simulink model "hcci_eng"  (R2018a)
settings: Solver=VariableStepAuto  StartTime=0.0  StopTime=10.0  RelTol=1e-3
values from neighbouring files (symbols this model uses):
  A01 = ???    [hcci_sim.m]
  A20 = ???    [hcci_sim.m]
  A21 = ???    [hcci_sim.m]
  b1_0 = ???    [load_param.m]
  b2_0 = ???    [load_param.m]
  C_d = ???    [hcci_sim.m]
  dT_er2 = 75    [load_param.m]
  gamma = 1.4    [load_param.m]
  m1_0 = ???    [load_param.m]
  m2_0 = ???    [load_param.m]
  N = 1000    [hcci_sim.m]
  p0 = 1.01    [load_param.m]
  R = 296.25    [load_param.m]
  T1 = 90 + 273.15    (= 363.15)    [load_param.m]
  tau = 120 / N    (= 0.12)    [hcci_sim.m]
  V1 = ???    [load_param.m]
  V2 = ???    [load_param.m]
undefined symbols (not defined in the file or in its folder): p2_0
settings Model: Creator=Lenovo  LastModifiedBy=Lenovo

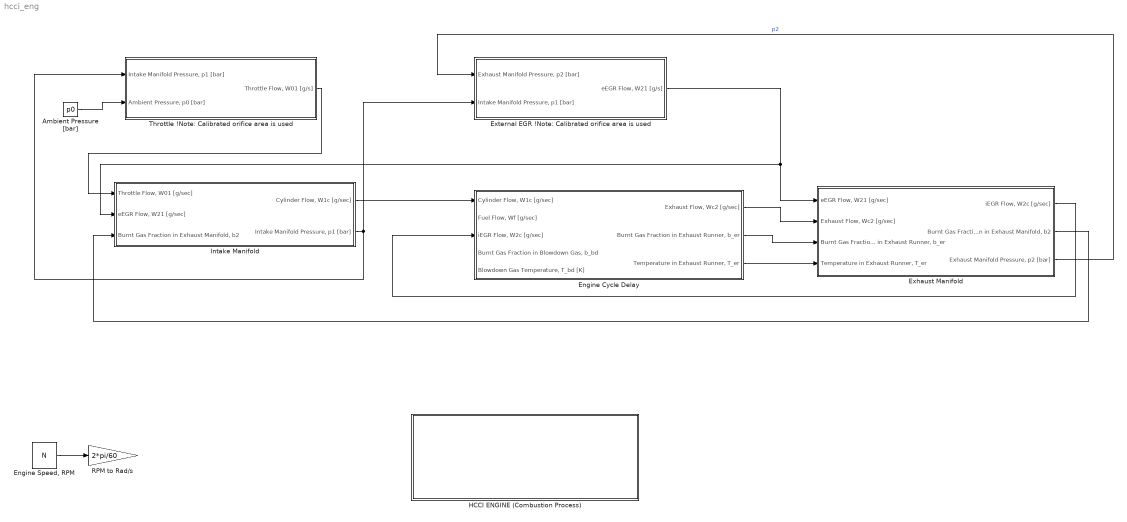
== system hcci_eng ==
  Ambient Pressure [bar] : Constant  Value=p0
  Engine Cycle Delay : Subsystem
  "Engine Speed, RPM" : Constant  Value=N
  Exhaust Manifold : Subsystem
  "External EGR !Note: Calibrated orifice area is used " : Subsystem
  HCCI ENGINE (Combustion Process) : Subsystem
  Intake Manifold : Subsystem
  RPM to Rad/s : Gain  Gain=2*pi/60
  Throttle !Note: Calibrated orifice area is used : Subsystem
  wires:
  "Engine Speed, RPM"/1 -> RPM to Rad/s/1
  Ambient Pressure [bar]/1 -> Throttle !Note: Calibrated orifice area is used/2("Ambient Pressure, p0 [bar]")
  Throttle !Note: Calibrated orifice area is used/1("Throttle Flow, W01 [g/s]") -> Intake Manifold/1("Throttle Flow, W01 [g/sec]")
  Intake Manifold/2("Intake Manifold Pressure, p1 [bar]") -> "External EGR !Note: Calibrated orifice area is used "/2("Intake Manifold Pressure, p1 [bar]"), Throttle !Note: Calibrated orifice area is used/1("Intake Manifold Pressure, p1 [bar]")
  "External EGR !Note: Calibrated orifice area is used "/1("eEGR Flow, W21 [g/s]") -> Exhaust Manifold/1("eEGR Flow, W21 [g/sec]"), Intake Manifold/2("eEGR Flow, W21 [g/sec]")
  Exhaust Manifold/2("Burnt Gas Fraction in Exhaust Manifold, b2") -> Intake Manifold/3("Burnt Gas Fraction in Exhaust Manifold, b2")
  Intake Manifold/1("Cylinder Flow, W1c [g/sec]") -> Engine Cycle Delay/1("Cylinder Flow, W1c [g/sec]")
  Exhaust Manifold/1("iEGR Flow, W2c [g/sec]") -> Engine Cycle Delay/3("iEGR Flow, W2c [g/sec]")
  Engine Cycle Delay/1("Exhaust Flow, Wc2 [g/sec]") -> Exhaust Manifold/2("Exhaust Flow, Wc2 [g/sec]")
  Engine Cycle Delay/2("Burnt Gas Fraction in Exhaust Runner, b_er") -> Exhaust Manifold/3("Burnt Gas Fraction in Exhaust Runner, b_er")
  Engine Cycle Delay/3("Temperature in Exhaust Runner, T_er") -> Exhaust Manifold/4("Temperature in Exhaust Runner, T_er")
  Exhaust Manifold/3("Exhaust Manifold Pressure, p2 [bar]") -> "External EGR !Note: Calibrated orifice area is used "/1("Exhaust Manifold Pressure, p2 [bar]")  "p2"

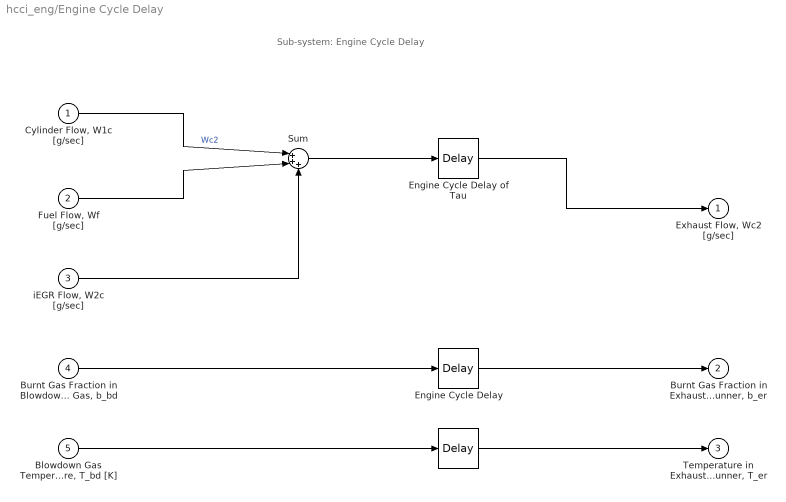
== system hcci_eng/Engine Cycle Delay ==
  note: Sub-system: Engine Cycle Delay
  "Cylinder Flow, W1c [g/sec]" : Inport
  "Fuel Flow, Wf [g/sec]" : Inport  Port=2
  "iEGR Flow, W2c [g/sec]" : Inport  Port=3
  "Burnt Gas Fraction in Blowdown Gas, b_bd " : Inport  Port=4
  "Blowdown Gas Temperature, T_bd [K]" : Inport  Port=5
  " " : TransportDelay  DelayTime=tau
  Engine Cycle Delay : TransportDelay  DelayTime=tau
  Engine Cycle Delay of Tau : TransportDelay  DelayTime=tau
  Sum : Sum  Inputs=|+++
  "Exhaust Flow, Wc2 [g/sec]" : Outport
  "Burnt Gas Fraction in Exhaust Runner, b_er" : Outport  Port=2
  "Temperature in Exhaust Runner, T_er" : Outport  Port=3
  wires:
  "Cylinder Flow, W1c [g/sec]"/1 -> Sum/1  "Wc2"
  "Fuel Flow, Wf [g/sec]"/1 -> Sum/2
  "iEGR Flow, W2c [g/sec]"/1 -> Sum/3
  Sum/1 -> Engine Cycle Delay of Tau/1
  Engine Cycle Delay of Tau/1 -> "Exhaust Flow, Wc2 [g/sec]"/1
  "Blowdown Gas Temperature, T_bd [K]"/1 -> " "/1
  "Burnt Gas Fraction in Blowdown Gas, b_bd "/1 -> Engine Cycle Delay/1
  " "/1 -> "Temperature in Exhaust Runner, T_er"/1
  Engine Cycle Delay/1 -> "Burnt Gas Fraction in Exhaust Runner, b_er"/1

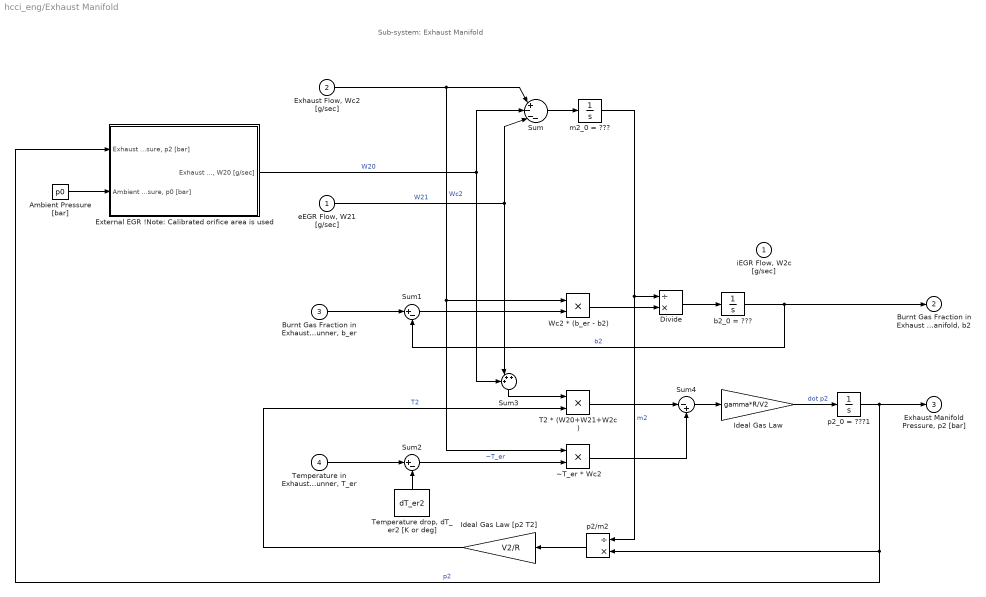
== system hcci_eng/Exhaust Manifold ==
  note: Sub-system: Exhaust Manifold
  "eEGR Flow, W21 [g/sec]" : Inport
  "Exhaust Flow, Wc2 [g/sec]" : Inport  Port=2
  "Burnt Gas Fraction in Exhaust Runner, b_er" : Inport  Port=3
  "Temperature in Exhaust Runner, T_er" : Inport  Port=4
  Ambient Pressure [bar] : Constant  Value=p0
  Divide : Product  Inputs=/*
  "External EGR !Note: Calibrated orifice area is used " : Subsystem
  Ideal Gas Law : Gain  Gain=gamma*R/V2
  Ideal Gas Law [p2 T2] : Gain  Gain=V2/R
  Sum : Sum  Inputs=|+---
  Sum1 : Sum  Inputs=|+-
  Sum2 : Sum  Inputs=|+-
  Sum3 : Sum  Inputs=+++|
  Sum4 : Sum  Inputs=|-+
  T2 * (W20+W21+W2c) : Product
  "Temperature drop, dT_er2 [K or deg] " : Constant  Value=dT_er2
  Wc2 * (b_er - b2) : Product
  b2_0 = ??? : Integrator  InitialCondition=b2_0
  m2_0 = ??? : Integrator  InitialCondition=m2_0
  p2/m2 : Product  Inputs=/*
  p2_0 = ???1 : Integrator  InitialCondition=p2_0
  ~T_er * Wc2 : Product
  "iEGR Flow, W2c [g/sec]" : Outport
  "Burnt Gas Fraction in Exhaust Manifold, b2" : Outport  Port=2
  "Exhaust Manifold Pressure, p2 [bar]" : Outport  Port=3
  wires:
  "Exhaust Flow, Wc2 [g/sec]"/1 -> Sum/1, Wc2 * (b_er - b2)/1, ~T_er * Wc2/1  "Wc2"
  "External EGR !Note: Calibrated orifice area is used "/1("Exhaust Flow, W20 [g/sec]") -> Sum/2, Sum3/1  "W20"
  "eEGR Flow, W21 [g/sec]"/1 -> Sum3/2, Sum/3  "W21"
  ? -> Sum3/3, Sum/4, "iEGR Flow, W2c [g/sec]"/1  "W2c"
  Sum/1 -> m2_0 = ???/1
  m2_0 = ???/1 -> p2/m2/1, Divide/1  "m2"
  Divide/1 -> b2_0 = ???/1
  Wc2 * (b_er - b2)/1 -> Divide/2
  b2_0 = ???/1 -> "Burnt Gas Fraction in Exhaust Manifold, b2"/1, Sum1/2  "b2"
  "Burnt Gas Fraction in Exhaust Runner, b_er"/1 -> Sum1/1
  Sum1/1 -> Wc2 * (b_er - b2)/2
  "Temperature in Exhaust Runner, T_er"/1 -> Sum2/1
  "Temperature drop, dT_er2 [K or deg] "/1 -> Sum2/2
  Sum2/1 -> ~T_er * Wc2/2  "~T_er"
  Sum3/1 -> T2 * (W20+W21+W2c)/1
  Ideal Gas Law [p2 T2]/1 -> T2 * (W20+W21+W2c)/2  "T2"
  T2 * (W20+W21+W2c)/1 -> Sum4/1
  ~T_er * Wc2/1 -> Sum4/2
  Sum4/1 -> Ideal Gas Law/1
  Ideal Gas Law/1 -> p2_0 = ???1/1  "dot p2"
  p2_0 = ???1/1 -> "Exhaust Manifold Pressure, p2 [bar]"/1, "External EGR !Note: Calibrated orifice area is used "/1("Exhaust Manifold Pressure, p2 [bar]"), p2/m2/2  "p2"
  p2/m2/1 -> Ideal Gas Law [p2 T2]/1
  Ambient Pressure [bar]/1 -> "External EGR !Note: Calibrated orifice area is used "/2("Ambient Pressure, p0 [bar]")

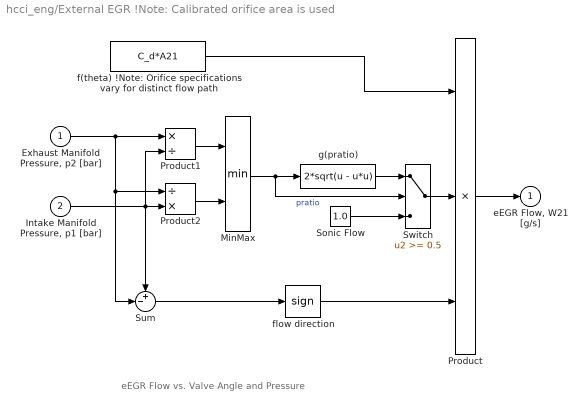
== system hcci_eng/External EGR !Note: Calibrated orifice area is used  ==
  note: eEGR Flow vs. Valve Angle and Pressure
  "Exhaust Manifold Pressure, p2 [bar]" : Inport
  "Intake Manifold Pressure, p1 [bar]" : Inport  Port=2
  MinMax : MinMax  Inputs=2  SaturateOnIntegerOverflow=on  InputSameDT=on
  Product : Product  Inputs=3  SaturateOnIntegerOverflow=on  RndMeth=Zero  InputSameDT=on  OutDataTypeStr=Inherit: Same as first input
  Product1 : Product  Inputs=*/  SaturateOnIntegerOverflow=on  RndMeth=Zero  InputSameDT=on  OutDataTypeStr=Inherit: Same as first input
  Product2 : Product  Inputs=/*  SaturateOnIntegerOverflow=on  RndMeth=Zero  InputSameDT=on  OutDataTypeStr=Inherit: Same as first input
  "Sonic Flow " : Constant  Value=1.0
  Sum : Sum  Inputs=+-|  SaturateOnIntegerOverflow=on  InputSameDT=on  OutDataTypeStr=Inherit: Same as first input
  Switch : Switch  Threshold=0.5  SaturateOnIntegerOverflow=on  InputSameDT=on
  "f(theta) !Note: Orifice specifications vary for distinct flow path " : Constant  Value=C_d*A21
  flow direction : Signum
  g(pratio) : Fcn  Expr=2*sqrt(u - u*u)
  "eEGR Flow, W21 [g/s]" : Outport  InitialOutput=0
  wires:
  "Exhaust Manifold Pressure, p2 [bar]"/1 -> Sum/2, Product2/1, Product1/1
  Product2/1 -> MinMax/2
  Product1/1 -> MinMax/1
  "Intake Manifold Pressure, p1 [bar]"/1 -> Sum/1, Product2/2, Product1/2
  g(pratio)/1 -> Switch/1
  "Sonic Flow "/1 -> Switch/3
  Switch/1 -> Product/2
  flow direction/1 -> Product/3
  Sum/1 -> flow direction/1
  MinMax/1 -> Switch/2, g(pratio)/1  "pratio"
  Product/1 -> "eEGR Flow, W21 [g/s]"/1
  "f(theta) !Note: Orifice specifications vary for distinct flow path "/1 -> Product/1

== system hcci_eng/HCCI ENGINE (Combustion Process) ==
  note: HCCI ENGINE: Combustion MVM

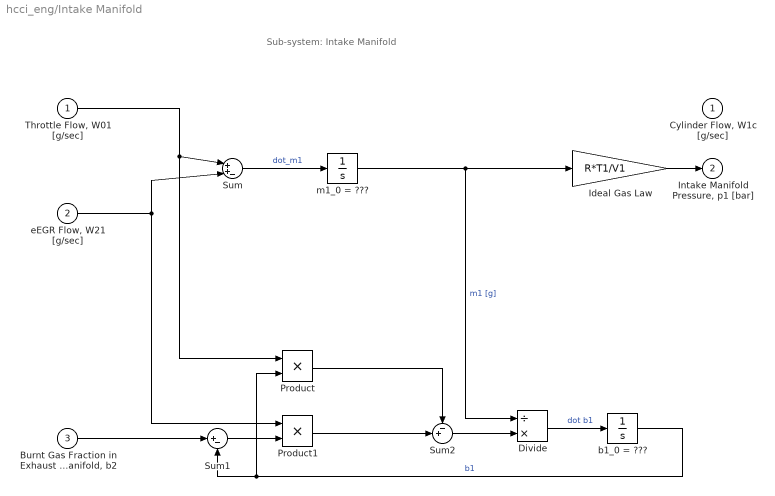
== system hcci_eng/Intake Manifold ==
  note: Sub-system: Intake Manifold
  "Throttle Flow, W01 [g/sec]" : Inport
  "eEGR Flow, W21 [g/sec]" : Inport  Port=2
  "Burnt Gas Fraction in Exhaust Manifold, b2" : Inport  Port=3
  Divide : Product  Inputs=/*
  Ideal Gas Law : Gain  Gain=R*T1/V1
  Product : Product
  Product1 : Product
  Sum : Sum  Inputs=|++-
  Sum1 : Sum  Inputs=|+-
  Sum2 : Sum  Inputs=-+|
  b1_0 = ??? : Integrator  InitialCondition=b1_0
  m1_0 = ??? : Integrator  InitialCondition=m1_0
  "Cylinder Flow, W1c [g/sec]" : Outport
  "Intake Manifold Pressure, p1 [bar]" : Outport  Port=2
  wires:
  ? -> Sum/3  "W1c"
  "Throttle Flow, W01 [g/sec]"/1 -> Product/1, Sum/1
  "eEGR Flow, W21 [g/sec]"/1 -> Product1/1, Sum/2
  Sum/1 -> m1_0 = ???/1  "dot_m1"
  m1_0 = ???/1 -> Ideal Gas Law/1, Divide/1  "m1 [g]"
  "Burnt Gas Fraction in Exhaust Manifold, b2"/1 -> Sum1/1
  Sum1/1 -> Product1/2
  Product1/1 -> Sum2/2
  Product/1 -> Sum2/1
  Sum2/1 -> Divide/2
  Divide/1 -> b1_0 = ???/1  "dot b1"
  b1_0 = ???/1 -> Product/2, Sum1/2  "b1"
  Ideal Gas Law/1 -> "Intake Manifold Pressure, p1 [bar]"/1
  ? -> "Cylinder Flow, W1c [g/sec]"/1

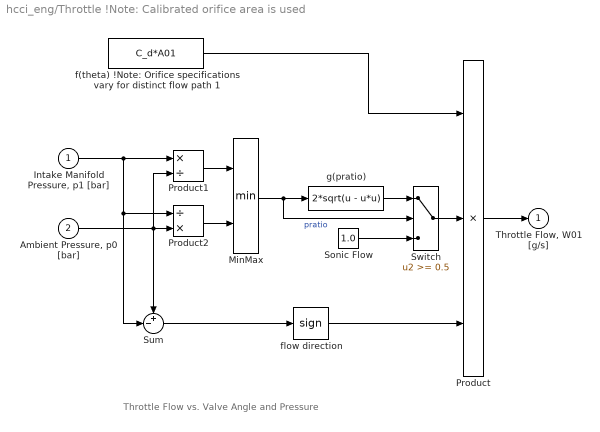
== system hcci_eng/Throttle !Note: Calibrated orifice area is used ==
  note: Throttle Flow vs. Valve Angle and Pressure
  "Intake Manifold Pressure, p1 [bar]" : Inport
  "Ambient Pressure, p0 [bar]" : Inport  Port=2
  MinMax : MinMax  Inputs=2  SaturateOnIntegerOverflow=on  InputSameDT=on
  Product : Product  Inputs=3  SaturateOnIntegerOverflow=on  RndMeth=Zero  InputSameDT=on  OutDataTypeStr=Inherit: Same as first input
  Product1 : Product  Inputs=*/  SaturateOnIntegerOverflow=on  RndMeth=Zero  InputSameDT=on  OutDataTypeStr=Inherit: Same as first input
  Product2 : Product  Inputs=/*  SaturateOnIntegerOverflow=on  RndMeth=Zero  InputSameDT=on  OutDataTypeStr=Inherit: Same as first input
  "Sonic Flow " : Constant  Value=1.0
  Sum : Sum  Inputs=+-|  SaturateOnIntegerOverflow=on  InputSameDT=on  OutDataTypeStr=Inherit: Same as first input
  Switch : Switch  Threshold=0.5  SaturateOnIntegerOverflow=on  InputSameDT=on
  f(theta) !Note: Orifice specifications vary for distinct flow path 1 : Constant  Value=C_d*A01
  flow direction : Signum
  g(pratio) : Fcn  Expr=2*sqrt(u - u*u)
  "Throttle Flow, W01 [g/s]" : Outport  InitialOutput=0
  wires:
  "Intake Manifold Pressure, p1 [bar]"/1 -> Sum/2, Product2/1, Product1/1
  Product2/1 -> MinMax/2
  Product1/1 -> MinMax/1
  "Ambient Pressure, p0 [bar]"/1 -> Sum/1, Product2/2, Product1/2
  g(pratio)/1 -> Switch/1
  "Sonic Flow "/1 -> Switch/3
  Switch/1 -> Product/2
  flow direction/1 -> Product/3
  Sum/1 -> flow direction/1
  MinMax/1 -> Switch/2, g(pratio)/1  "pratio"
  Product/1 -> "Throttle Flow, W01 [g/s]"/1
  f(theta) !Note: Orifice specifications vary for distinct flow path 1/1 -> Product/1

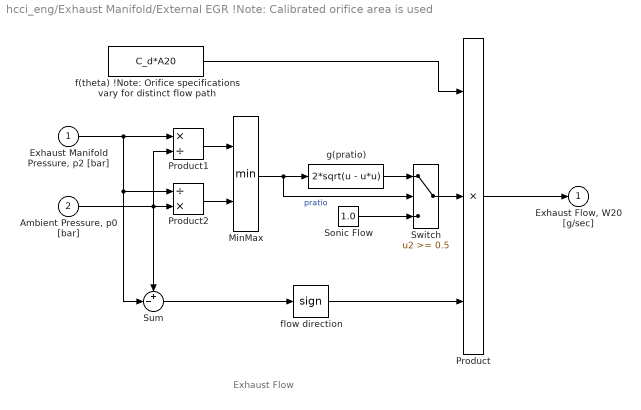
== system hcci_eng/Exhaust Manifold/External EGR !Note: Calibrated orifice area is used  ==
  note: Exhaust Flow
  "Exhaust Manifold Pressure, p2 [bar]" : Inport
  "Ambient Pressure, p0 [bar]" : Inport  Port=2
  MinMax : MinMax  Inputs=2  SaturateOnIntegerOverflow=on  InputSameDT=on
  Product : Product  Inputs=3  SaturateOnIntegerOverflow=on  RndMeth=Zero  InputSameDT=on  OutDataTypeStr=Inherit: Same as first input
  Product1 : Product  Inputs=*/  SaturateOnIntegerOverflow=on  RndMeth=Zero  InputSameDT=on  OutDataTypeStr=Inherit: Same as first input
  Product2 : Product  Inputs=/*  SaturateOnIntegerOverflow=on  RndMeth=Zero  InputSameDT=on  OutDataTypeStr=Inherit: Same as first input
  "Sonic Flow " : Constant  Value=1.0
  Sum : Sum  Inputs=+-|  SaturateOnIntegerOverflow=on  InputSameDT=on  OutDataTypeStr=Inherit: Same as first input
  Switch : Switch  Threshold=0.5  SaturateOnIntegerOverflow=on  InputSameDT=on
  "f(theta) !Note: Orifice specifications vary for distinct flow path " : Constant  Value=C_d*A20
  flow direction : Signum
  g(pratio) : Fcn  Expr=2*sqrt(u - u*u)
  "Exhaust Flow, W20 [g/sec]" : Outport  InitialOutput=0
  wires:
  "Exhaust Manifold Pressure, p2 [bar]"/1 -> Sum/2, Product2/1, Product1/1
  Product2/1 -> MinMax/2
  Product1/1 -> MinMax/1
  "Ambient Pressure, p0 [bar]"/1 -> Sum/1, Product2/2, Product1/2
  g(pratio)/1 -> Switch/1
  "Sonic Flow "/1 -> Switch/3
  Switch/1 -> Product/2
  flow direction/1 -> Product/3
  Sum/1 -> flow direction/1
  MinMax/1 -> Switch/2, g(pratio)/1  "pratio"
  Product/1 -> "Exhaust Flow, W20 [g/sec]"/1
  "f(theta) !Note: Orifice specifications vary for distinct flow path "/1 -> Product/1
